simulink model "foreach"  (R2023b)
settings: Solver=FixedStepDiscrete  StartTime=0.0  StopTime=10.0  RelTol=1e-3
settings Model: SimulationMode=accelerator  Creator=mfussi  LastModifiedBy=mfussi
settings OptimizationCC: DefaultParameterBehavior=Inlined  EnhancedBackFolding=on  PassReuseOutputArgsAs=Individual arguments  ZeroExternalMemoryAtStartup=off  ZeroInternalMemoryAtStartup=off  OptimizeBlockOrder=speed  DifferentSizesBufferReuse=on  OptimizationCustomize=off  EfficientTunableParamExpr=on
settings DebuggingCC: ParameterTunabilityLossMsg=error
settings SFSimCC: MATLABDynamicMemAlloc=off
settings RTWCC: Description=Embedded Coder  SystemTargetFile=ert.tlc  TemplateMakefile=ert_default_tmf
settings CodeAppCC: ForceParamTrailComments=on  IgnoreCustomStorageClasses=off  OperatorAnnotations=on  SimulinkDataObjDesc=on  SFDataObjDesc=on  InsertBlockDesc=on
settings ERTTargetCC: TargetLangStandard=C99 (ISO)  GenerateSampleERTMain=on  InlinedParameterPlacement=NonHierarchical  ERTCustomFileTemplate=example_file_process.tlc

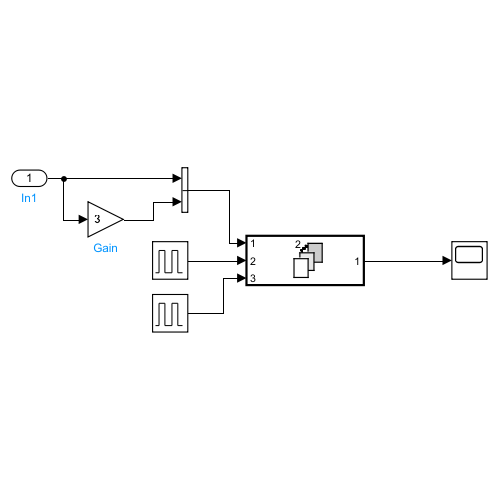
[thumbnail: Simulink's stored preview of the top-level diagram]
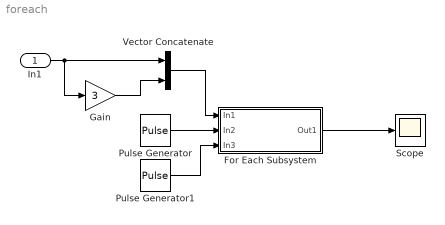
== system foreach ==
  In1 : Inport
  For Each Subsystem : Subsystem  TreatAsAtomicUnit=on
  Gain : Gain  Gain=3
  Pulse Generator : DiscretePulseGenerator  PulseType=Time based  Period=1  PulseWidth=50
  Pulse Generator1 : DiscretePulseGenerator  PulseType=Time based  Period=1  PulseWidth=5  PhaseDelay=0.75
  Scope : Scope
  Vector Concatenate : Concatenate
  wires:
  Vector Concatenate/1 -> For Each Subsystem/1(In1)
  In1/1 -> Gain/1, Vector Concatenate/1
  Gain/1 -> Vector Concatenate/2
  For Each Subsystem/1(Out1) -> Scope/1
  Pulse Generator/1 -> For Each Subsystem/2(In2)
  Pulse Generator1/1 -> For Each Subsystem/3(In3)

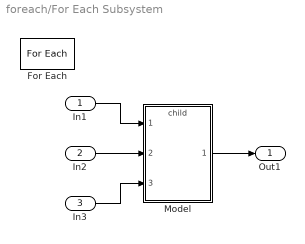
== system foreach/For Each Subsystem ==
  In1 : Inport  Partition=on  PartitionDimension=1  PartitionWidth=1  PartitionOffset=0
  In2 : Inport  Port=2
  In3 : Inport  Port=3
  For Each : ForEach  DisableCoverage=on
  Model : ModelReference  ModelNameDialog=child.slx  ModelReferenceVersion=1.11
  Out1 : Outport  ConcatenationDimension=1
  wires:
  In1/1 -> Model/1
  Model/1 -> Out1/1
  In2/1 -> Model/2
  In3/1 -> Model/3
